simulink model "ObtenerDatosSensores_Harness1"  (R2020b)
settings: Solver=VariableStepAuto  StartTime=0.0  StopTime=10.0  RelTol=1e-3
settings Model: Creator=sergi  LastModifiedBy=sergi

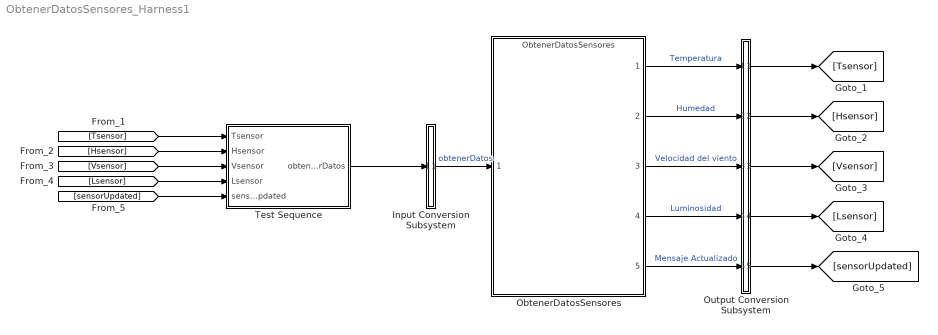
== system ObtenerDatosSensores_Harness1 ==
  Input Conversion Subsystem : Subsystem  Tag=__SLT_ICS__  Description=|
      | Signal spec.
      | and routing
      settings: AttributesFormatString=%<Description>
  ObtenerDatosSensores : ModelReference  ModelNameDialog=ObtenerDatosSensores  SimulationMode=Normal  ModelReferenceVersion=1.38
  Output Conversion Subsystem : Subsystem  Tag=__SLT_OCS__  Description=|
      | Signal spec.
      | and routing
      settings: AttributesFormatString=%<Description>
  Test Sequence : Test Sequence  TreatAsAtomicUnit=on
  wires:
  Test Sequence/1(obtenerDatos) -> Input Conversion Subsystem/1(Inport_1)
  [Tsensor] -> Test Sequence/1(Tsensor)
  [Hsensor] -> Test Sequence/2(Hsensor)
  [Vsensor] -> Test Sequence/3(Vsensor)
  [Lsensor] -> Test Sequence/4(Lsensor)
  [sensorUpdated] -> Test Sequence/5(sensorUpdated)
  Output Conversion Subsystem/1(Outport_1) -> [Tsensor]
  Output Conversion Subsystem/2(Outport_2) -> [Hsensor]
  Output Conversion Subsystem/3(Outport_3) -> [Vsensor]
  Output Conversion Subsystem/4(Outport_4) -> [Lsensor]
  Output Conversion Subsystem/5(Outport_5) -> [sensorUpdated]
  Input Conversion Subsystem/1(Outport_1) -> ObtenerDatosSensores/1  "obtenerDatos"
  ObtenerDatosSensores/1 -> Output Conversion Subsystem/1(Inport_1)  "Temperatura"
  ObtenerDatosSensores/2 -> Output Conversion Subsystem/2(Inport_2)  "Humedad"
  ObtenerDatosSensores/3 -> Output Conversion Subsystem/3(Inport_3)  "Velocidad del viento"
  ObtenerDatosSensores/4 -> Output Conversion Subsystem/4(Inport_4)  "Luminosidad"
  ObtenerDatosSensores/5 -> Output Conversion Subsystem/5(Inport_5)  "Mensaje Actualizado"

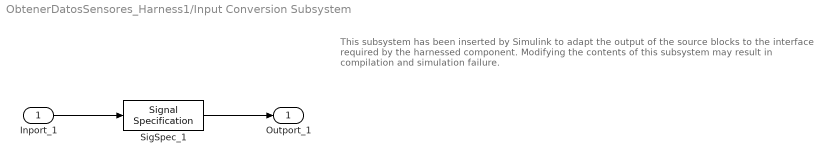
== system ObtenerDatosSensores_Harness1/Input Conversion Subsystem ==
  note: This subsystem has been inserted by Simulink to adapt the output of the source blocks to the interface required by the harnessed component.
      |  Modifying the contents of this subsystem may result in compilation and simulation failure.
  Inport_1 : Inport
  SigSpec_1 : SignalSpecification  OutDataTypeStr=double  Dimensions=[1]  SampleTime=[-1, 0]
  Outport_1 : Outport
  wires:
  SigSpec_1/1 -> Outport_1/1
  Inport_1/1 -> SigSpec_1/1

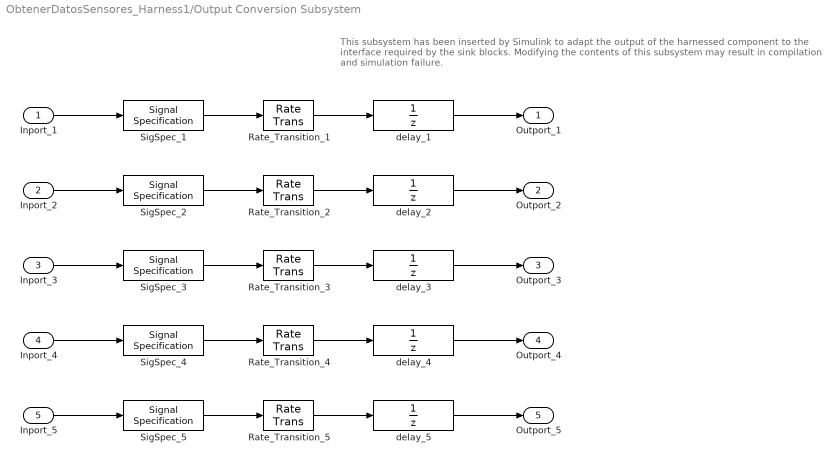
== system ObtenerDatosSensores_Harness1/Output Conversion Subsystem ==
  note: This subsystem has been inserted by Simulink to adapt the output of the harnessed component to the interface required by the sink blocks.
      |  Modifying the contents of this subsystem may result in compilation and simulation failure.
  Inport_1 : Inport
  Inport_2 : Inport  Port=2
  Inport_3 : Inport  Port=3
  Inport_4 : Inport  Port=4
  Inport_5 : Inport  Port=5
  Rate_Transition_{1..5} (5 alike) : RateTransition  OutPortSampleTimeOpt=Inherit
  SigSpec_{1..5} (5 alike) : SignalSpecification  OutDataTypeStr=double  Dimensions=[1]  SampleTime=0.2
  delay_{1..5} (5 alike) : UnitDelay  SampleTime=-1
  Outport_1 : Outport
  Outport_2 : Outport  Port=2
  Outport_3 : Outport  Port=3
  Outport_4 : Outport  Port=4
  Outport_5 : Outport  Port=5
  wires:
  Inport_1/1 -> SigSpec_1/1
  SigSpec_1/1 -> Rate_Transition_1/1
  Rate_Transition_1/1 -> delay_1/1
  delay_1/1 -> Outport_1/1
  Inport_2/1 -> SigSpec_2/1
  SigSpec_2/1 -> Rate_Transition_2/1
  Rate_Transition_2/1 -> delay_2/1
  delay_2/1 -> Outport_2/1
  Inport_3/1 -> SigSpec_3/1
  SigSpec_3/1 -> Rate_Transition_3/1
  Rate_Transition_3/1 -> delay_3/1
  delay_3/1 -> Outport_3/1
  Inport_4/1 -> SigSpec_4/1
  SigSpec_4/1 -> Rate_Transition_4/1
  Rate_Transition_4/1 -> delay_4/1
  delay_4/1 -> Outport_4/1
  Inport_5/1 -> SigSpec_5/1
  SigSpec_5/1 -> Rate_Transition_5/1
  Rate_Transition_5/1 -> delay_5/1
  delay_5/1 -> Outport_5/1

== stateflow chart ObtenerDatosSensores_Harness1/Test Sequence ==
  settings: stateMachineType=SIMPLIFIED_MACHINE
  state Run
    %% Initialize data outputs.
    obtenerDatos = 0;
  state step_1
    obtenerDatos = 1;
  state step_2
    obtenerDatos = 0;
  (default) -> Run
  (junction 31) -> Run
  (junction 33) -> (junction 31)
  Run -> step_1 : [
      | after(0.1,sec)
      | ]
  step_1 -> step_2 : [
      | after(2,sec)
      | ]
  step_2 -> (junction 33) : [
      | after(0.1,sec)
      | ]
  data: Tsensor input double size=[1]; Hsensor input double size=[1]; Vsensor input double size=[1]; Lsensor input double size=[1]; sensorUpdated input double size=[1]; obtenerDatos output double size=[1]
